simulink model "pato04"  (Simulink 4.00)
settings: Solver=ode1  StartTime=0.0  StopTime=3600  FixedStep=1/4096  RelTol=1e-3
settings Model: Creator=root  LastModifiedBy=root  MaxDataPoints=4000*3600  SimulationMode=external  RTWSystemTargetFile=wintarget.tlc  RTWOptions="-aEnforceIntegerDowncast=1 -aExtMode=1 -aFoldNonRolledExpr=1 -aForceParamTrailComments=0 -aGenerateComments=1 -aIgnoreCustomStorageClasses=1 -aIncHierarchyInIds=0 -aInlineInvariantSignals=0 -aInlineParameters=0 -aLocalBlockOutputs=1 -aLogVarNameModifier=\"rt_\" -aRTWVerbose=1 -aRollThreshold=5 -aShowEliminatedStatements=1"  RTWTemplateMakefile=wt_default_tmf  ExtModeTrigElement=1  ExtModeTrigDuration=3910  ExtModeAutoUpdateStatusClock=off  BlockReductionOpt=off

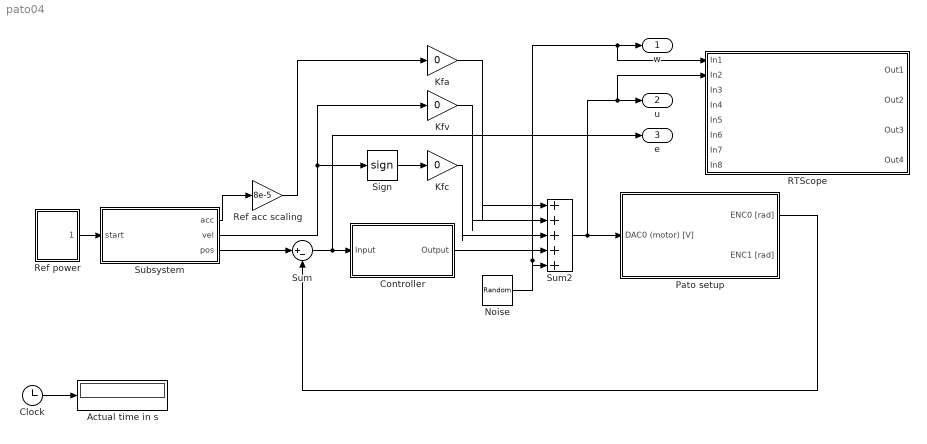
== system pato04 ==
  Actual time in s : Display
      settings: Format=short
  Clock : Clock
      settings: DisplayTime=off  Decimation=10
  Controller : Subsystem  mask(Controller){Kp=2, Kv=.01, notch_zeros=300, notch_damping_zeros=0.1, notch_poles=300, notch_damping_poles=0.1, roll_off_poles=300, roll_off_damping_poles=0.2}
      mask prompts: notch_zeros "Notch zeros [Hz]"; notch_damping_zeros "Notch damping zeros [-]"; notch_poles "Notch poles [Hz]"; notch_damping_poles "Notch damping poles [-]"; roll_off_poles "Roll-off poles [Hz]"; roll_off_damping_poles "Roll-off damping poles [-]"
      mask help:
      | The controller consists of three filters: a Kp/Kv, a notch and a roll-off filter.
      | You can edit the parameters below.
      settings: RTWFcnNameOpts=Auto  RTWFileNameOpts=Auto
  Kfa : Gain  Gain=0  Multiplication=Element-wise(K.*u)  SaturateOnIntegerOverflow=on
  Kfc : Gain  Gain=0  Multiplication=Element-wise(K.*u)  SaturateOnIntegerOverflow=on
  Kfv : Gain  Gain=0  Multiplication=Element-wise(K.*u)  SaturateOnIntegerOverflow=on
  Noise : RandomNumber  Mean=0  Variance=0.2  Seed=0  SampleTime=0
  Pato setup : Subsystem
      settings: RTWFcnNameOpts=Auto  RTWFileNameOpts=Auto
      mask Type: Encoders
      mask Description: Inc encoder positions 1-2 [rad] (see connector pannel).
  RTScope : Subsystem
      settings: OpenFcn=rtscope  RTWFcnNameOpts=Auto  RTWFileNameOpts=Auto
      mask Type: RTScope
      mask Display: image(imread('rtscope2.jpg'))
  "Ref acc scaling " : Gain  Gain=8e-5  Multiplication=Element-wise(K.*u)  SaturateOnIntegerOverflow=on
  Ref power : Subsystem  mask(On/Off Switch){stat=Off}
      mask prompts: stat "Switch"
      settings: RTWFcnNameOpts=Auto  RTWFileNameOpts=Auto
      mask StyleString: popup(On|Off)
  Sign : Signum
  Subsystem : Subsystem
      settings: OpenFcn=global ref_part; cb_axes 1  RTWFcnNameOpts=Auto  RTWFileNameOpts=Auto
      mask Type: Ref3
      mask Display: disp('Ref3');
  Sum : Sum  Inputs=|+-  SaturateOnIntegerOverflow=on
  Sum2 : Sum  Description=sumff  Inputs=|+++++  SaturateOnIntegerOverflow=on
  w : Outport  Port=1
  u : Outport  Port=2
  e : Outport  Port=3
  wires:
  "Ref acc scaling "/1 -> Kfa/1
  Sum/1 -> Controller/1(Input), e/1
  Controller/1(Output) -> Sum2/4
  Sign/1 -> Kfc/1
  Kfc/1 -> Sum2/3
  Kfv/1 -> Sum2/2
  Kfa/1 -> Sum2/1
  Ref power/1(On/Off) -> Subsystem/1(start)
  Sum2/1 -> Pato setup/1(DAC0 (motor) [V]), u/1, RTScope/2(In2)
  Pato setup/1(ENC0 [rad]) -> Sum/2
  Noise/1 -> Sum2/5, w/1, RTScope/1(In1)
  Subsystem/1(acc) -> "Ref acc scaling "/1
  Subsystem/3(pos) -> Sum/1
  Subsystem/2(vel) -> Kfv/1, Sign/1
  Clock/1 -> Actual time in s/1

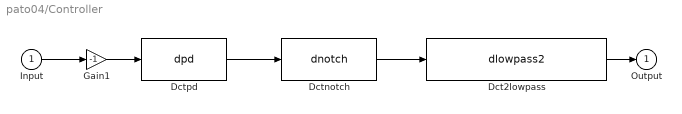
== system pato04/Controller ==
  Input : Inport  Port=1  LatchInput=off
  Dct2lowpass : S-Function  FunctionName=dlowpass2  Parameters=[f_den b_den 0.001]  PortCounts=[]  SFunctionModules=''  mask(dctools){f_den=roll_off_poles, b_den=roll_off_damping_poles}
      mask prompts: f_den "Pole [Hz]"; b_den "Damping pole [-]"
      mask help: This block implements a discrete time 2nd order lowpass filter.
      mask Display: disp('DCT 2nd order lowpass')
  Dctnotch : S-Function  FunctionName=dnotch  Parameters=[f_num b_num f_den b_den 0.001]  PortCounts=[]  SFunctionModules=''  mask(dctools){f_num=notch_zeros, b_num=notch_damping_zeros, f_den=notch_poles, b_den=notch_damping_poles}
      mask prompts: f_num "Zero [Hz]"; b_num "Damping zero [-]"; f_den "Pole [Hz]"; b_den "Damping pole [-]"
      mask help: This block implements a dicrete time 2nd order notch filter.
      mask Display: disp('DCT notch')
  Dctpd : S-Function  FunctionName=dpd  Parameters=[kp kv 0.001]  PortCounts=[]  SFunctionModules=''  mask(dctools){kp=Kp, kv=Kv}
      mask help: This block implements a discrete time pd filter.
      mask Display: disp('DCT pd')
  Gain1 : Gain  Gain=-1  Multiplication=Element-wise(K.*u)  SaturateOnIntegerOverflow=on
  Output : Outport  Port=1
  wires:
  Dct2lowpass/1 -> Output/1
  Gain1/1 -> Dctpd/1
  Input/1 -> Gain1/1
  Dctpd/1 -> Dctnotch/1
  Dctnotch/1 -> Dct2lowpass/1

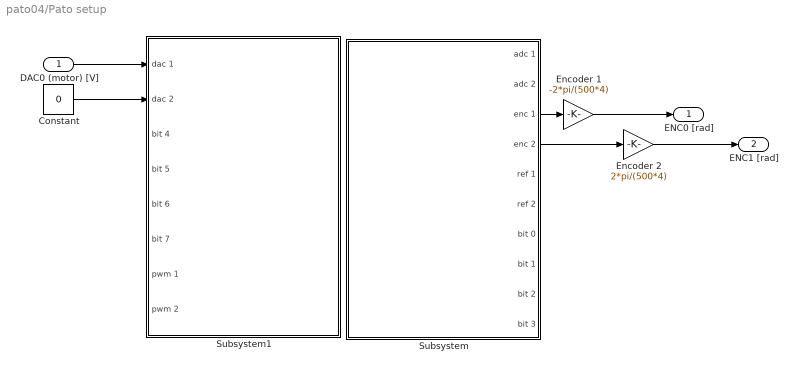
== system pato04/Pato setup ==
  DAC0 (motor) [V] : Inport  Port=1  LatchInput=off
  Constant : Constant  Value=0
  Encoder 1 : Gain  Gain=-2*pi/(500*4)  Multiplication=Element-wise(K.*u)  SaturateOnIntegerOverflow=on
  Encoder 2 : Gain  Gain=2*pi/(500*4)  Multiplication=Element-wise(K.*u)  SaturateOnIntegerOverflow=on
  Subsystem : Subsystem  mask(TUeDACS/1 QAD/AQI Inports block){ilink=link0, adc_active_ch1=off, adc_range_select_ch1=+/- 10 V, adc_active_ch2=off, adc_range_select_ch2=+/- 10 V, enc_active_ch1=on, enc_funct_select_ch1=Quadrature single ended, enc_active_ch2=on, enc_funct_select_ch2=Quadrature single ended, dio_active=off}
      mask prompts: ilink "QAD/AQI identifier"; adc_active_ch1 "Use ADC channel 1"; adc_range_select_ch1 "ADC range select channel 1 (AQI only)"; adc_active_ch2 "Use ADC channel 2"; adc_range_select_ch2 "ADC range select channel 2 (AQI only)"; enc_active_ch1 "Use ENC channel 1"; enc_funct_select_ch1 "ENC function select channel 1"; enc_active_ch2 "Use ENC channel 2"; enc_funct_select_ch2 "ENC function select channel 2"; dio_active "Use DI channels"
      mask help:
      | This block models the TUeDACS/1 QAD/AQI inports.
      |
      | QAD:
      | - front panel channels are named 0/1 instead of 1/2
      | - ADC input range is fixed at +/- 2.5 V
      |
      | AQI:
      | - scalable ADC input range
      settings: RTWFcnNameOpts=Auto  RTWFileNameOpts=Auto
      mask Help: This block models the TUeDACS/1 QAD/AQI inports.
      mask StyleString: popup(link0|link1),checkbox,popup(+/- 10 V|+/- 5 V|+/- 2 V|+/- 1 V|+/- 0.5 V|+/- 0.2 V|+/- 0.1 V),checkbox,popup(+/- 10 V|+/- 5 V|+/- 2 V|+/- 1 V|+/- 0.5 V|+/- 0.2 V|+/- 0.1 V),checkbox,popup(Quadrature single ended|Quadrature differential (AQI only)|Event counter),checkbox,popup(Quadrature single ended|Quadrature differential (AQI only)|Event counter),checkbox
      mask Display:
      | disp('TUeDACS/1 QAD/AQI');
      | disp('\n\nInports block');
  Subsystem1 : Subsystem  mask(TUeDACS/1 QAD/AQI Outports block){ilink=link0, dac_active_ch1=on, dac_hold_order_select_ch1=Zero order (SW), dac_active_ch2=off, dac_hold_order_select_ch2=Zero order (SW), dio_active=off, pwm_active_ch1=off, pwm_funct_select_ch1=Locked anti-phase PWM (0 to 1), pwm_freq_select_ch1=10 kHz, pwm_active_ch2=off, pwm_funct_select_ch2=Locked anti-phase PWM (0 to 1), pwm_freq_select_ch2=10 kHz}
      mask prompts: ilink "QAD/AQI identifier"; dac_active_ch1 "Use DAC channel 1"; dac_hold_order_select_ch1 "DAC hold order select channel 1"; dac_active_ch2 "Use DAC channel 2"; dac_hold_order_select_ch2 "DAC hold order select channel 2"; dio_active "Use DO channels"; pwm_active_ch1 "Use PWM channel 1 (AQI only)"; pwm_funct_select_ch1 "PWM function select channel 1"; pwm_freq_select_ch1 "PWM frequency select channel 1"; pwm_active_ch2 "Use PWM channel 2 (AQI only)"; pwm_funct_select_ch2 "PWM function select channel 2"; pwm_freq_select_ch2 "PWM frequency select channel 2"
      mask help:
      | This block models the TUeDACS/1 QAD/AQI outports.
      |
      | QAD:
      | - front panel channels are named 0/1 instead of 1/2
      | - DAC output range is +/- 2.5 V
      |
      | AQI:
      | - DAC output range is +/- 5V.
      | - scalable ADC input range
      settings: RTWFcnNameOpts=Auto  RTWFileNameOpts=Auto
      mask Help: This block models the TUeDACS/1 QAD/AQI outports.
      mask StyleString: popup(link0|link1),checkbox,popup(Zero order (SW)|First order (SW)|Second order (SW)|Third order (SW)),checkbox,popup(Zero order (SW)|First order (SW)|Second order (SW)|Third order (SW)),checkbox,checkbox,popup(Locked anti-phase PWM (0 to 1)|Sign/magnitude PWM (-1 to 1)),popup(1 Hz|10 Hz|50 Hz|100 Hz|1 kHz|10 kHz|100 kHz|1 MHz),checkbox,popup(Locked anti-phase PWM (0 to 1)|Sign/magnitude PWM (-1 to 1)),popup(1 Hz|10 Hz|50 Hz|100 Hz|1 kHz|10 kHz|100 kHz|1 MHz)
      mask Display:
      | disp('TUeDACS/1 QAD/AQI');
      | disp('\n\nOutports block');
  ENC0 [rad] : Outport  Port=1
  ENC1 [rad] : Outport  Port=2
  wires:
  Subsystem/3(enc 1) -> Encoder 1/1
  Encoder 1/1 -> ENC0 [rad]/1
  Encoder 2/1 -> ENC1 [rad]/1
  DAC0 (motor) [V]/1 -> Subsystem1/1(dac 1)
  Subsystem/4(enc 2) -> Encoder 2/1
  Constant/1 -> Subsystem1/2(dac 2)

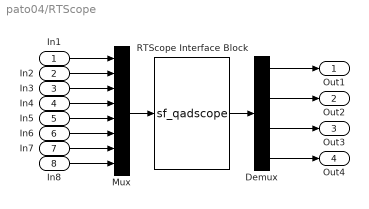
== system pato04/RTScope ==
  In1 : Inport  Port=1  LatchInput=off
  In2 : Inport  Port=2  LatchInput=off
  In3 : Inport  Port=3  LatchInput=off
  In4 : Inport  Port=4  LatchInput=off
  In5 : Inport  Port=5  LatchInput=off
  In6 : Inport  Port=6  LatchInput=off
  In7 : Inport  Port=7  LatchInput=off
  In8 : Inport  Port=8  LatchInput=off
  Demux : Demux  Outputs=4  BusSelectionMode=off
  Mux : Mux  Inputs=8
  RTScope Interface Block : S-Function  FunctionName=sf_qadscope  Parameters=4000  PortCounts=[]  SFunctionModules=''
      settings: OpenFcn=rtscope
  Out1 : Outport  Port=1
  Out2 : Outport  Port=2
  Out3 : Outport  Port=3
  Out4 : Outport  Port=4
  wires:
  In8/1 -> Mux/8
  In7/1 -> Mux/7
  In6/1 -> Mux/6
  In5/1 -> Mux/5
  In4/1 -> Mux/4
  In3/1 -> Mux/3
  In2/1 -> Mux/2
  In1/1 -> Mux/1
  Demux/4 -> Out4/1
  Demux/3 -> Out3/1
  Demux/2 -> Out2/1
  Demux/1 -> Out1/1
  RTScope Interface Block/1 -> Demux/1
  Mux/1 -> RTScope Interface Block/1

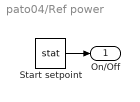
== system pato04/Ref power ==
  Start setpoint : Constant  Value=stat
  On/Off : Outport  Port=1
  wires:
  Start setpoint/1 -> On/Off/1

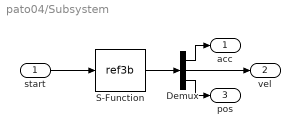
== system pato04/Subsystem ==
  start : Inport  Port=1  LatchInput=off
  Demux : Demux  Outputs=3  BusSelectionMode=off
  S-Function : S-Function  FunctionName=ref3b  Parameters=ref_part  PortCounts=[]  SFunctionModules=''
      settings: OpenFcn=global ref_part; r3g_main
  acc : Outport  Port=1
  vel : Outport  Port=2
  pos : Outport  Port=3
  wires:
  S-Function/1 -> Demux/1
  Demux/1 -> acc/1
  Demux/2 -> vel/1
  Demux/3 -> pos/1
  start/1 -> S-Function/1

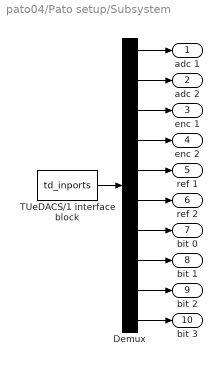
== system pato04/Pato setup/Subsystem ==
  Demux : Demux  Outputs=10  BusSelectionMode=off
  TUeDACS/1 interface block : S-Function  FunctionName=td_inports  Parameters=ilink, adc_active_ch1, adc_active_ch2, enc_active_ch1, enc_active_ch2, dio_active, adc_range_select_ch1, adc_range_select_ch2, enc_funct_select_ch1, enc_funct_select_ch2  PortCounts=[]  SFunctionModules=''
  adc 1 : Outport  Port=1
  adc 2 : Outport  Port=2
  enc 1 : Outport  Port=3
  enc 2 : Outport  Port=4
  ref 1 : Outport  Port=5
  ref 2 : Outport  Port=6
  bit 0 : Outport  Port=7
  bit 1 : Outport  Port=8
  bit 2 : Outport  Port=9
  bit 3 : Outport  Port=10
  wires:
  TUeDACS/1 interface block/1 -> Demux/1
  Demux/1 -> adc 1/1
  Demux/2 -> adc 2/1
  Demux/3 -> enc 1/1
  Demux/4 -> enc 2/1
  Demux/7 -> bit 0/1
  Demux/8 -> bit 1/1
  Demux/9 -> bit 2/1
  Demux/10 -> bit 3/1
  Demux/5 -> ref 1/1
  Demux/6 -> ref 2/1

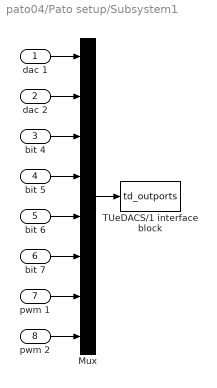
== system pato04/Pato setup/Subsystem1 ==
  dac 1 : Inport  Port=1  LatchInput=off
  dac 2 : Inport  Port=2  LatchInput=off
  bit 4 : Inport  Port=3  LatchInput=off
  bit 5 : Inport  Port=4  LatchInput=off
  bit 6 : Inport  Port=5  LatchInput=off
  bit 7 : Inport  Port=6  LatchInput=off
  pwm 1 : Inport  Port=7  LatchInput=off
  pwm 2 : Inport  Port=8  LatchInput=off
  Mux : Mux  Inputs=8
  TUeDACS/1 interface block : S-Function  FunctionName=td_outports  Parameters=ilink, dac_active_ch1, dac_hold_order_select_ch1, dac_active_ch2, dac_hold_order_select_ch2, dio_active, pwm_active_ch1, pwm_active_ch2, pwm_funct_select_ch1, pwm_funct_select_ch2, pwm_freq_select_ch1, pwm_freq_select_ch2  PortCounts=[]  SFunctionModules=''
  wires:
  Mux/1 -> TUeDACS/1 interface block/1
  dac 1/1 -> Mux/1
  dac 2/1 -> Mux/2
  bit 4/1 -> Mux/3
  bit 5/1 -> Mux/4
  bit 6/1 -> Mux/5
  bit 7/1 -> Mux/6
  pwm 2/1 -> Mux/8
  pwm 1/1 -> Mux/7
